simulink library "Tire_MFSwift"  (R2019a)
settings: Solver=VariableStepAuto  StartTime=0.0  StopTime=10.0  RelTol=1e-3
undefined symbols (not defined in the file): Left, UNLOADED_RADIUS, Vehicle, VERTICAL_DAMPING, VERTICAL_STIFFNESS, Visual, X, Y, Z
libraries: nesl_utility x24, sm_lib x15, mfswift_simscape_library x2, Delft_Tyre_dtlib x1, TireBody_Models x1, sm_car_lib x1, $bdroot x1
(part 2 of 2)

== system Tire_MFSwift/CPI Tire/Tire and Force ==
  Inertia : sm_lib/Body Elements/Solid  InertiaType=Custom  Mass=mass  MassUnits=kg  CenterOfMass=[0 0 0]  CenterOfMassUnits=m  MomentsOfInertia=[Imat(1,1) Imat(2,2) Imat(3,3)]  MomentsOfInertiaUnits=kg*m^2  ProductsOfInertia=[0 0 0]  ProductsOfInertiaUnits=kg*m^2  BasedOnType=Density  Density=1000  DensityUnits=kg/(m^3)  DoExposeReferenceFrame=on  SerializedFrames=<Frames/>  GraphicType=FromGeometry  MarkerShape=Sphere  MarkerSize=10  MarkerSizeUnits=m  GraphicVisPropType=SimpleVisualProperties  GraphicDiffuseColor=[0.2 0.8 1.0]  GraphicSpecularColor=[0.5 0.5 0.5 1.0]  GraphicAmbientColor=[0.15 0.15 0.15 1.0]  GraphicEmissiveColor=[0.0 0.0 0.0 1.0]  GraphicShininess=75  GraphicOpacity=1.0  GeometryShape=Cylinder  RectangleSize=[1 1]  RectangleSizeUnits=m  BrickDimensions=[3 1 0.5]  BrickDimensionUnits=m  CylinderRadius=0.001  CylinderRadiusUnits=m  CylinderLength=0.001  CylinderLengthUnits=m  SphereRadius=0.001  SphereRadiusUnits=m  EllipsoidRadii=[1 1 1]  EllipsoidRadiiUnits=m  ExtrusionCrossSection=[1 1; -1 1; -1 -1; 1 -1]  ExtrusionCrossSectionUnits=m  ExtrusionLength=1  ExtrusionLengthUnits=m  PolygonNumSides=3  PolygonOuterRadius=1  PolygonOuterRadiusUnits=m  ExtGeomFileType=STEP  ExtGeomFileName=.\CadImportFiles\Tire.STL  ExtGeomFileUnits=mm  RevolutionCrossSection=[1 1; 1 -1; 2 -1; 2 1]  RevolutionCrossSectionUnits=m  RevolutionExtent=Full  RevolutionAngle=180  RevolutionAngleUnits=deg
  Rim : sm_lib/Body Elements/Solid  InertiaType=Custom  Mass=0  MassUnits=kg  CenterOfMass=[0 0 0]  CenterOfMassUnits=m  MomentsOfInertia=[0 0 0]  MomentsOfInertiaUnits=kg*m^2  ProductsOfInertia=[0 0 0]  ProductsOfInertiaUnits=kg*m^2  BasedOnType=Density  Density=1000  DensityUnits=kg/(m^3)  DoExposeReferenceFrame=on  SerializedFrames=<Frames/>  GraphicType=FromGeometry  MarkerShape=Sphere  MarkerSize=10  MarkerSizeUnits=m  GraphicVisPropType=SimpleVisualProperties  GraphicDiffuseColor=clr_rim_cfl  GraphicSpecularColor=[0.5 0.5 0.5 1.0]  GraphicAmbientColor=[0.15 0.15 0.15 1.0]  GraphicEmissiveColor=[0.0 0.0 0.0 1.0]  GraphicShininess=75  GraphicOpacity=opc_rim_cfl  GeometryShape=RegularExtrusion  RectangleSize=[1 1]  RectangleSizeUnits=m  BrickDimensions=[1 1 1]  BrickDimensionUnits=m  CylinderRadius=1  CylinderRadiusUnits=m  CylinderLength=1  CylinderLengthUnits=m  SphereRadius=1  SphereRadiusUnits=m  EllipsoidRadii=[1 1 1]  EllipsoidRadiiUnits=m  ExtrusionCrossSection=[1 1; -1 1; -1 -1; 1 -1]  ExtrusionCrossSectionUnits=m  ExtrusionLength=width*0.1  ExtrusionLengthUnits=m  PolygonNumSides=5  PolygonOuterRadius=rim_radius  PolygonOuterRadiusUnits=m  ExtGeomFileType=STL  ExtGeomFileName=Rim.STL  ExtGeomFileUnits=mm  RevolutionCrossSection=[1 1; 1 -1; 2 -1; 2 1]  RevolutionCrossSectionUnits=m  RevolutionExtent=Full  RevolutionAngle=180  RevolutionAngleUnits=deg
  Tire : sm_lib/Body Elements/Solid  InertiaType=Custom  Mass=0  MassUnits=kg  CenterOfMass=[0 0 0]  CenterOfMassUnits=m  MomentsOfInertia=[0 0 0]  MomentsOfInertiaUnits=kg*m^2  ProductsOfInertia=[0 0 0]  ProductsOfInertiaUnits=kg*m^2  BasedOnType=Density  Density=1000  DensityUnits=kg/(m^3)  DoExposeReferenceFrame=on  SerializedFrames=<Frames/>  GraphicType=FromGeometry  MarkerShape=Sphere  MarkerSize=10  MarkerSizeUnits=m  GraphicVisPropType=SimpleVisualProperties  GraphicDiffuseColor=clr_tyre_cfl  GraphicSpecularColor=[0.5 0.5 0.5 1.0]  GraphicAmbientColor=[0.15 0.15 0.15 1.0]  GraphicEmissiveColor=[0.0 0.0 0.0 1.0]  GraphicShininess=75  GraphicOpacity=opc_tyre_cfl  GeometryShape=GeneralSolidOfRevolution  RectangleSize=[1 1]  RectangleSizeUnits=m  BrickDimensions=[1 1 1]  BrickDimensionUnits=m  CylinderRadius=1  CylinderRadiusUnits=m  CylinderLength=1  CylinderLengthUnits=m  SphereRadius=1  SphereRadiusUnits=m  EllipsoidRadii=[1 1 1]  EllipsoidRadiiUnits=m  ExtrusionCrossSection=[1 1; -1 1; -1 -1; 1 -1]  ExtrusionCrossSectionUnits=m  ExtrusionLength=1  ExtrusionLengthUnits=m  PolygonNumSides=3  PolygonOuterRadius=1  PolygonOuterRadiusUnits=m  ExtGeomFileType=STL  ExtGeomFileName=Tire.STL  ExtGeomFileUnits=mm  RevolutionCrossSection="[1  0.5; rim_radius/radius 0.5; rim_radius/radius -0.5; 1 -0.5].*[radius  width]"  RevolutionCrossSectionUnits=m  RevolutionExtent=Full  RevolutionAngle=180  RevolutionAngleUnits=deg
  Transform Geometry : sm_lib/Frames and Transforms/Rigid Transform  TranslationMethod=StandardAxis  TranslationStandardOffset=0  TranslationLengthUnit=m  TranslationStandardAxis=+Y  TranslationCartesianOffset=[0 0 0]  TranslationROffset=0  TranslationROffsetUnits=m  TranslationZOffset=0  TranslationZOffsetUnits=m  TranslationThetaOffset=0  TranslationThetaOffsetUnits=deg  RotationMethod=StandardAxis  RotationAngleUnits=deg  RotationStandardAxis=+X  RotationAngle=-90  RotationArbitraryAxis=[0 0 1]  FollAlignAxisA=+X  BaseAlignAxisA=+Y  FollAlignAxisB=+Y  BaseAlignAxisB=+Z  RotationSequenceAxes=FollowerAxes  RotationSequence=XYX  RotationSequenceAngles=[0 0 0]  RotationSequenceAnglesUnits=deg  RotationMatrix=[1 0 0; 0 1 0; 0 0 1]
  Transform Spin Axis : sm_lib/Frames and Transforms/Rigid Transform  TranslationMethod=None  TranslationStandardOffset=0  TranslationLengthUnit=m  TranslationStandardAxis=+Z  TranslationCartesianOffset=[0 0 0]  TranslationROffset=0  TranslationROffsetUnits=m  TranslationZOffset=0  TranslationZOffsetUnits=m  TranslationThetaOffset=0  TranslationThetaOffsetUnits=deg  RotationMethod=StandardAxis  RotationAngleUnits=deg  RotationStandardAxis=-X  RotationAngle=90  RotationArbitraryAxis=[0 0 1]  FollAlignAxisA=+X  BaseAlignAxisA=+Y  FollAlignAxisB=+Y  BaseAlignAxisB=+Z  RotationSequenceAxes=FollowerAxes  RotationSequence=XYX  RotationSequenceAngles=[0 0 0]  RotationSequenceAnglesUnits=deg  RotationMatrix=[1 0 0; 0 1 0; 0 0 1]
  B : PMIOPort  Side=Left
  connections:
  Transform Spin Axis/RConn1 -- B/RConn1
  Tire/RConn1 -- Transform Geometry/RConn1 -- Inertia/RConn1 -- Rim/RConn1
  Transform Spin Axis/LConn1 -- Transform Geometry/LConn1

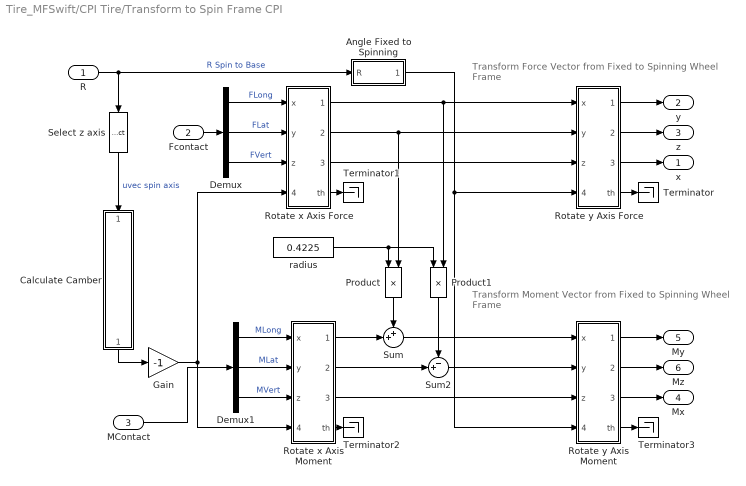
== system Tire_MFSwift/CPI Tire/Transform to Spin Frame CPI ==
  note: Transform Moment Vector from Fixed
      | to Spinning Wheel Frame
  note: Transform Force Vector from Fixed
      | to Spinning Wheel Frame
  R : Inport
  Fcontact : Inport  Port=2
  MContact : Inport  Port=3
  Angle Fixed to Spinning : Subsystem
  Calculate Camber : Subsystem
  Demux : Demux  Outputs=3
  Demux1 : Demux  Outputs=3
  Gain : Gain  Gain=-1
  Product : Product
  Product1 : Product
  Rotate x Axis Force : Subsystem
  Rotate x Axis Moment : Subsystem
  Rotate y Axis Force : Subsystem
  Rotate y Axis Moment : Subsystem
  Select z axis : Selector  NumberOfDimensions=2  InputPortWidth=2  IndexOptions=Index vector (dialog),Index vector (dialog)  Indices=[1 2 3],3  OutputSizes=1,1
  Sum : Sum  Inputs=++|
  Sum2 : Sum  Inputs=-+|
  Terminator{,1..3} (4 alike) : Terminator
  radius : Constant  Value=0.4225
  x : Outport
  y : Outport  Port=2
  z : Outport  Port=3
  Mx : Outport  Port=4
  My : Outport  Port=5
  Mz : Outport  Port=6
  wires:
  R/1 -> Select z axis/1, Angle Fixed to Spinning/1(R)  "R Spin to Base"
  Angle Fixed to Spinning/1(rotang) -> Rotate y Axis Moment/4(theta), Rotate y Axis Force/4(theta)
  Rotate y Axis Moment/1(x rot) -> My/1
  Rotate y Axis Moment/2(y rot) -> Mz/1
  Rotate x Axis Moment/1(x rot) -> Sum/2
  Rotate x Axis Force/1(x rot) -> Product1/2, Rotate y Axis Force/1(x)
  Rotate y Axis Force/1(x rot) -> y/1
  Rotate y Axis Force/2(y rot) -> z/1
  Select z axis/1 -> Calculate Camber/1(uvec spin axis)  "uvec spin axis"
  Demux/1 -> Rotate x Axis Force/1(x)  "FLong"
  Demux/3 -> Rotate x Axis Force/3(z)  "FVert"
  Calculate Camber/1(Camber) -> Gain/1
  Demux1/3 -> Rotate x Axis Moment/3(z)  "MVert"
  Demux1/1 -> Rotate x Axis Moment/1(x)  "MLong"
  Demux1/2 -> Rotate x Axis Moment/2(y)  "MLat"
  Product/1 -> Sum/1
  radius/1 -> Product1/1, Product/1
  Rotate x Axis Force/3(z rot) -> Rotate y Axis Force/3(z)
  Product1/1 -> Sum2/1
  Demux/2 -> Rotate x Axis Force/2(y)  "FLat"
  Rotate x Axis Force/2(y rot) -> Rotate y Axis Force/2(y), Product/2
  Rotate y Axis Force/3(z rot) -> x/1
  Rotate y Axis Force/4(th) -> Terminator/1
  Rotate x Axis Force/4(th) -> Terminator1/1
  Rotate x Axis Moment/2(y rot) -> Sum2/2
  Rotate x Axis Moment/4(th) -> Terminator2/1
  Rotate y Axis Moment/3(z rot) -> Mx/1
  Rotate y Axis Moment/4(th) -> Terminator3/1
  Sum2/1 -> Rotate y Axis Moment/2(y)
  Sum/1 -> Rotate y Axis Moment/1(x)
  Rotate x Axis Moment/3(z rot) -> Rotate y Axis Moment/3(z)
  Gain/1 -> Rotate x Axis Force/4(theta), Rotate x Axis Moment/4(theta)
  Fcontact/1 -> Demux/1
  MContact/1 -> Demux1/1

== system Tire_MFSwift/CPI Tire/Vertical Force ==
  camber : Inport
  h : Inport  Port=2
  vz : Inport  Port=3
  gz : Inport  Port=4
  Constant1 : Constant  Value=UNLOADED_RADIUS
  Cos : Trigonometry  Operator=cos
  Damping Force : Subsystem
  Product : Product
  Subtract : Sum  Inputs=+-
  Sum : Sum  Inputs=|+-
  Sum1 : Sum  Inputs=|+-
  Tire Vertical Stiffness : Lookup_n-D  NumberOfTableDimensions=1  BreakpointsForDimension1=[-1 0 0.1]  Table=[VERTICAL_STIFFNESS 0 0]  InternalRulePriority=Speed  RndMeth=Simplest  InputSameDT=on
  Fvert : Outport
  wires:
  h/1 -> Subtract/1
  Sum1/1 -> Fvert/1
  camber/1 -> Cos/1
  gz/1 -> Sum/2
  Cos/1 -> Product/2
  vz/1 -> Damping Force/2(vz)
  Subtract/1 -> Sum/1
  Damping Force/1(Fz d) -> Sum1/2
  Product/1 -> Subtract/2
  Sum/1 -> Tire Vertical Stiffness/1
  Constant1/1 -> Product/1
  Tire Vertical Stiffness/1 -> Damping Force/1(Fz k), Sum1/1

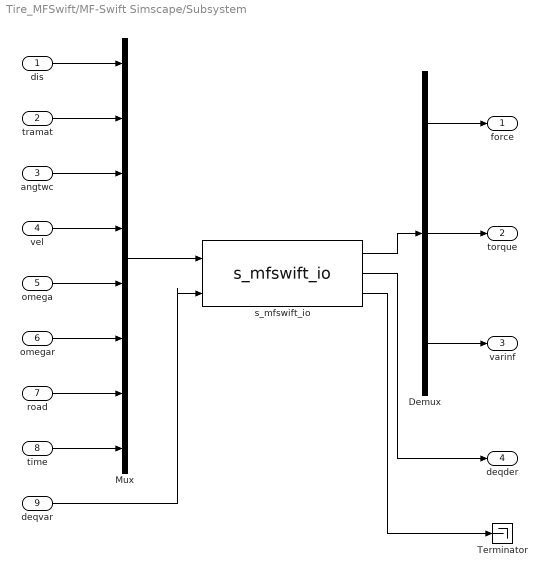
== system Tire_MFSwift/MF-Swift Simscape/Subsystem ==
  dis : Inport
  tramat : Inport  Port=2
  angtwc : Inport  Port=3
  vel : Inport  Port=4
  omega : Inport  Port=5
  omegar : Inport  Port=6
  road : Inport  Port=7
  time : Inport  Port=8
  deqvar : Inport  Port=9
  Demux : Demux  Outputs=[3 3 60]
  Mux : Mux  Inputs=[3 9 1 3 3 1 20 1]
  Terminator : Terminator
  s_mfswift_io : S-Function  FunctionName=s_mfswift_io  Parameters=SParameter1, SParameter2, SParameter3, SParameter4, SParameter5,SParameter6,SParameter7  SFunctionDeploymentMode=off  EnableBusSupport=off  mask(Legacy Function){SFunctionSpec=tyre_outputs(void **work1, int32 p2, int16 p4[8], double u1[41], double u2[40], int16 work2[1], double work3[1], double y1[66], double y2[40], int16 y3[1]), SParameter1=iswtch, SParameter2=idtyre, SParameter3=typarr, SParameter4=uint8([tyreSimulationMode 0]), SParameter5=uint8([tyreTargetFile 0]), SParameter6=uint8([tyreTemplateMakefile 0]), SParameter7=roadfile, ShowSpec=off}
      mask prompts: SParameter1 "P1: iswtch"; SParameter2 "P2: idtyre"; SParameter3 "P3: typarr"; SParameter4 "P4: simulation mode"; SParameter5 "P5: target file"; SParameter6 "P6: template makefile"; SParameter7 "P7: road file name"; ShowSpec "Display function specification"
      mask help:
      | This block allows you to call the legacy functions specified by the following Legacy Code Tool definition:
      | def.SFunctionName = 's_mfswift_io';
      | def.OutputFcnSpec = 'tyre_outputs(void **work1, int32 p2, int16 p4[8], double u1[41], double u2[40], int16 work2[1], double work3[1], double y1[66], double y2[40], int16 y3[1])';
      | def.StartFcnSpec = 'tyre_start(void **work1, int32 p1, int32 p2, double p3[300], int16 p4[8], uint8 p5[], int16 work2[1], double work3[1])';
      | def.TerminateFcnSpec = 'tyre_terminate(void **work1, int32 p2, int16 p4[8], int16 work2[1])';
      | def.HeaderFiles = {'tyremain.h', 'mfs_dtemsg.h'};
      | def.SourceFiles = {'dtemsg.c', 'console_writer.c'};
      | def.HostLibFiles = {'s_mfswift_io_impld.lib'};
      | def.TargetLibFiles = {'mfs_platform_generic_r2009a_ds1006.lib', 'mfs_kernel_r2009a_ds1006.lib', 'mfs_callback_r2009a_ds1006.lib', 'mfs_generic_r2009a_ds1006.lib', 'mfs_utilities_system_r2009a_ds1006.lib', 'mfs_platform_license_flexlm_r2009a_ds1006.lib', 'mfs_platform_license_stub_r2009a_ds1006.lib', 'mfs_log_r2009a_ds1006.lib'};
      | def.IncPaths = {'../headers'};
      | def.SrcPaths = {'../sources'};
      | def.LibPaths = {'../libraries/windows_win64', '../libraries/dSPACE_ds1006'};
      mask Help: <p>This block was generated automatically by the Legacy Code Tool. For detailed help on this tool, call<a href="matlab:legacy_code('help')"> legacy_code('help')</a>.</p>
      mask Callback ShowSpec:
      | if strcmp(get_param(gcbh, 'ShowSpec'), 'on')
      |   set_param(gcbh, 'MaskDisplay', sprintf('fprintf(''%s'');', get_param(gcbh, 'SFunctionSpec')));
      | else
      |   set_param(gcbh, 'MaskDisplay', sprintf('fprintf(''%s'');', get_param(gcbh, 'FunctionName')));
      | end
      mask Display: fprintf('s_mfswift_io');
  force : Outport  VectorParamsAs1DForOutWhenUnconnected=on
  torque : Outport  Port=2  VectorParamsAs1DForOutWhenUnconnected=on
  varinf : Outport  Port=3  VectorParamsAs1DForOutWhenUnconnected=on
  deqder : Outport  Port=4  VectorParamsAs1DForOutWhenUnconnected=on
  wires:
  tramat/1 -> Mux/2
  angtwc/1 -> Mux/3
  vel/1 -> Mux/4
  omega/1 -> Mux/5
  omegar/1 -> Mux/6
  road/1 -> Mux/7
  dis/1 -> Mux/1
  Demux/2 -> torque/1
  Demux/1 -> force/1
  Demux/3 -> varinf/1
  Mux/1 -> s_mfswift_io/1
  s_mfswift_io/1 -> Demux/1
  s_mfswift_io/2 -> deqder/1
  deqvar/1 -> s_mfswift_io/2
  time/1 -> Mux/8
  s_mfswift_io/3 -> Terminator/1

== system Tire_MFSwift/MF-Swift Simscape/add signal names ==
  In1 : Inport
  Added for future extension : Terminator
  Bus Creator : BusCreator  Inputs=40
  Demux1 : Demux  Outputs=[ones(1,40) -1]
  Out1 : Outport  VectorParamsAs1DForOutWhenUnconnected=on
  wires:
  Demux1/41 -> Added for future extension/1
  Demux1/40 -> Bus Creator/40  "eff_plane_banking"
  Demux1/39 -> Bus Creator/39  "eff_plane_curvature"
  Demux1/38 -> Bus Creator/38  "eff_plane_angle"
  Demux1/37 -> Bus Creator/37  "eff_plane_height"
  Demux1/36 -> Bus Creator/36  "nz"
  Demux1/35 -> Bus Creator/35  "ny"
  Demux1/34 -> Bus Creator/34  "nx"
  Demux1/33 -> Bus Creator/33  "zcp"
  Demux1/32 -> Bus Creator/32  "ycp"
  Demux1/31 -> Bus Creator/31  "xcp"
  Demux1/30 -> Bus Creator/30  "_e30"
  Demux1/29 -> Bus Creator/29  "_e29"
  Demux1/28 -> Bus Creator/28  "travelled_distance"
  Demux1/27 -> Bus Creator/27  "_e27"
  Demux1/26 -> Bus Creator/26  "_e26"
  Demux1/25 -> Bus Creator/25  "_e25"
  Demux1/24 -> Bus Creator/24  "psidot"
  Demux1/23 -> Bus Creator/23  "Vz"
  Demux1/22 -> Bus Creator/22  "Vsy"
  Demux1/21 -> Bus Creator/21  "Vsx"
  Demux1/20 -> Bus Creator/20  "relaxation_length_y"
  Demux1/19 -> Bus Creator/19  "relaxation_length_x"
  Demux1/18 -> Bus Creator/18  "mu_y"
  Demux1/17 -> Bus Creator/17  "mu_x"
  Demux1/16 -> Bus Creator/16  "pneumatic_trail"
  Demux1/15 -> Bus Creator/15  "contact_length"
  Demux1/14 -> Bus Creator/14  "vertical_deflection"
  Demux1/13 -> Bus Creator/13  "effective_rolling_radius"
  Demux1/12 -> Bus Creator/12  "_e12"
  Demux1/11 -> Bus Creator/11  "Vx"
  Demux1/10 -> Bus Creator/10  "turn_slip"
  Demux1/9 -> Bus Creator/9  "inclination_angle"
  Demux1/8 -> Bus Creator/8  "side_slip_angle"
  Demux1/7 -> Bus Creator/7  "longitudinal_slip"
  Demux1/6 -> Bus Creator/6  "Mz"
  Demux1/5 -> Bus Creator/5  "My"
  Demux1/4 -> Bus Creator/4  "Mx"
  Demux1/3 -> Bus Creator/3  "Fz"
  Demux1/2 -> Bus Creator/2  "Fy"
  Demux1/1 -> Bus Creator/1  "Fx"
  Bus Creator/1 -> Out1/1  "varinf"
  In1/1 -> Demux1/1

== system Tire_MFSwift/MFSwift/Road Inputs ==
  note: 1) Only subsystems can be added as variant choices at this level
      | 2) Blocks cannot be connected at this level as connectivity is
      | automatically determined at simulation, based on the active variant
  RdBus : Inport
  External Road : Subsystem  VariantControl=ExternalRoad
  Non-moving road : mfswift_simscape_library/Non-moving road  VariantControl=NonMoving  dummy=off
  Test Rig Post : Subsystem  VariantControl=TestRigPost
  road : Outport

== system Tire_MFSwift/CPI Tire/Sensing Wheel Fixed Frame/Ang Velocity Vector ==
  Mux : Mux  Inputs=3
  PS-Simulink Converter1 : nesl_utility/PS-Simulink Converter  PhysicalDomain=network_engine_domain  SubClassName=ps_output  LeftPortType=input  RightPortType=output  PseudoPeriodic=off  Frequencies=[]  Unit=1  AffineConversion=off
  PS-Simulink Converter2 : nesl_utility/PS-Simulink Converter  PhysicalDomain=network_engine_domain  SubClassName=ps_output  LeftPortType=input  RightPortType=output  PseudoPeriodic=off  Frequencies=[]  Unit=1  AffineConversion=off
  PS-Simulink Converter3 : nesl_utility/PS-Simulink Converter  PhysicalDomain=network_engine_domain  SubClassName=ps_output  LeftPortType=input  RightPortType=output  PseudoPeriodic=off  Frequencies=[]  Unit=rad/s  AffineConversion=off
  Scope : Scope
  wx : PMIOPort  Side=Left
  wy : PMIOPort  Port=2  Side=Left
  wz : PMIOPort  Port=3  Side=Left
  wxyz : Outport
  wires:
  PS-Simulink Converter1/1 -> Mux/1
  PS-Simulink Converter3/1 -> Mux/3
  PS-Simulink Converter2/1 -> Mux/2
  Mux/1 -> wxyz/1, Scope/1
  connections:
  PS-Simulink Converter2/LConn1 -- wy/RConn1
  wx/RConn1 -- PS-Simulink Converter1/LConn1
  wz/RConn1 -- PS-Simulink Converter3/LConn1

== system Tire_MFSwift/CPI Tire/Sensing Wheel Fixed Frame/Calculate Camber ==
  uvec spin axis : Inport
  Demux : Demux  Outputs=3
  Mux : Mux  Inputs=2
  Trigonometric Function1 : Trigonometry  Operator=atan2
  magnitude : Fcn  Expr=sqrt(u(1)*u(1)+u(2)*u(2))
  Camber : Outport
  wires:
  Demux/1 -> Mux/1
  uvec spin axis/1 -> Demux/1
  Trigonometric Function1/1 -> Camber/1
  Demux/3 -> Trigonometric Function1/1
  Mux/1 -> magnitude/1
  magnitude/1 -> Trigonometric Function1/2
  Demux/2 -> Mux/2

== system Tire_MFSwift/CPI Tire/Sensing Wheel Fixed Frame/Get uvec Yaw axis ==
  note: Make Unit Vector
  note: Obtain unit vector along vertical axis within tire plane (wheel yaw axis)
      | (World Z vector [0 0 1])  -  (z-component of unit vector along wheel spin axis)
      | normalize ([0 0 1] - ([0 0 1].*uvec spin axis)*uvec spin axis)
  zf : Inport
  Add : Sum
  Constant : Constant
  Demux : Demux  Outputs=3
  Divide : Product  Inputs=*/
  Gain2 : Gain  Gain=-1
  Mult : Product  Inputs=**
  Mult1 : Product  Inputs=**
  Mult2 : Product  Inputs=**
  Mux1 : Mux  Inputs=3
  magnitude : Fcn  Expr=sqrt(u(1)*u(1)+u(2)*u(2)+u(3)*u(3))
  u : Outport
  wires:
  Add/1 -> Mux1/3
  Demux/2 -> Mult1/1
  Mux1/1 -> magnitude/1, Divide/1  "u0"
  Mult2/1 -> Add/1
  Demux/1 -> Mult/1
  zf/1 -> Demux/1
  Demux/3 -> Gain2/1, Mult2/1
  Gain2/1 -> Mult2/2, Mult1/2, Mult/2
  Mult1/1 -> Mux1/2
  Mult/1 -> Mux1/1
  Constant/1 -> Add/2
  Divide/1 -> u/1
  magnitude/1 -> Divide/2

== system Tire_MFSwift/CPI Tire/Sensing Wheel Fixed Frame/Project onto Road Plane ==
  note: Normalize to create a unit vector
  note: Create unit vector in lateral direction from wheel on ground plane.
      |
      | This computation projects input vector v (along the wheel spin axis) onto the plane normal to the z axis.
  v : Inport
  Constant : Constant  Value=0
  Demux : Demux  Outputs=3
  Divide : Product  Inputs=*/
  Mux1 : Mux  Inputs=3
  Terminator : Terminator
  magnitude : Fcn  Expr=sqrt(u(1)*u(1)+u(2)*u(2))
  v proj : Outport
  wires:
  Mux1/1 -> Divide/1, magnitude/1
  Demux/2 -> Mux1/2
  Demux/1 -> Mux1/1
  Constant/1 -> Mux1/3
  Demux/3 -> Terminator/1
  v/1 -> Demux/1
  Divide/1 -> v proj/1
  magnitude/1 -> Divide/2

== system Tire_MFSwift/CPI Tire/Sensing Wheel Fixed Frame/Rot -90 deg about Z ==
  v : Inport
  Demux : Demux  Outputs=3
  Gain : Gain  Gain=-1
  Mux1 : Mux  Inputs=3
  v rot -z : Outport
  wires:
  Demux/1 -> Gain/1
  Mux1/1 -> v rot -z/1
  Demux/3 -> Mux1/3
  Gain/1 -> Mux1/2
  Demux/2 -> Mux1/1
  v/1 -> Demux/1

== system Tire_MFSwift/CPI Tire/Sensing Wheel Fixed Frame/Velocity Vector ==
  Mux : Mux  Inputs=3
  PS-Simulink Converter1 : nesl_utility/PS-Simulink Converter  PhysicalDomain=network_engine_domain  SubClassName=ps_output  LeftPortType=input  RightPortType=output  PseudoPeriodic=off  Frequencies=[]  Unit=1  AffineConversion=off
  PS-Simulink Converter2 : nesl_utility/PS-Simulink Converter  PhysicalDomain=network_engine_domain  SubClassName=ps_output  LeftPortType=input  RightPortType=output  PseudoPeriodic=off  Frequencies=[]  Unit=1  AffineConversion=off
  PS-Simulink Converter3 : nesl_utility/PS-Simulink Converter  PhysicalDomain=network_engine_domain  SubClassName=ps_output  LeftPortType=input  RightPortType=output  PseudoPeriodic=off  Frequencies=[]  Unit=1  AffineConversion=off
  vx : PMIOPort  Side=Left
  vy : PMIOPort  Port=2  Side=Left
  vz : PMIOPort  Port=3  Side=Left
  vxyz : Outport
  wires:
  PS-Simulink Converter1/1 -> Mux/1
  PS-Simulink Converter3/1 -> Mux/3
  PS-Simulink Converter2/1 -> Mux/2
  Mux/1 -> vxyz/1
  connections:
  PS-Simulink Converter2/LConn1 -- vy/RConn1
  vx/RConn1 -- PS-Simulink Converter1/LConn1
  vz/RConn1 -- PS-Simulink Converter3/LConn1

== system Tire_MFSwift/CPI Tire/Transform to Spin Frame CPI/Angle Fixed to Spinning ==
  R : Inport
  Atan2 : Trigonometry  Operator=atan2
  Demux1 : Demux  Outputs=3
  Get uvec Yaw axis : Subsystem
  Multiply : Product  Inputs=**  Multiplication=Matrix(*)
  Select z axis : Selector  NumberOfDimensions=2  InputPortWidth=2  IndexOptions=Index vector (dialog),Index vector (dialog)  Indices=[1 2 3],3  OutputSizes=1,1
  Terminator : Terminator
  Transpose : Math  Operator=transpose  SaturateOnIntegerOverflow=on
  rotang : Outport
  wires:
  Demux1/2 -> Atan2/1
  Get uvec Yaw axis/1(u) -> Multiply/2  "Yaw vec Base"
  Demux1/1 -> Atan2/2
  Demux1/3 -> Terminator/1
  Select z axis/1 -> Get uvec Yaw axis/1(zf)  "uvec spin axis"
  R/1 -> Select z axis/1, Transpose/1
  Atan2/1 -> rotang/1
  Multiply/1 -> Demux1/1  "yaw vec spin frame"
  Transpose/1 -> Multiply/1  "R Base 2 Spin Frame"

== system Tire_MFSwift/CPI Tire/Transform to Spin Frame CPI/Calculate Camber ==
  uvec spin axis : Inport
  Demux : Demux  Outputs=3
  Mux : Mux  Inputs=2
  Trigonometric Function1 : Trigonometry  Operator=atan2
  magnitude : Fcn  Expr=sqrt(u(1)*u(1)+u(2)*u(2))
  Camber : Outport
  wires:
  Demux/2 -> Mux/2
  magnitude/1 -> Trigonometric Function1/2
  Mux/1 -> magnitude/1
  Demux/3 -> Trigonometric Function1/1
  Trigonometric Function1/1 -> Camber/1
  uvec spin axis/1 -> Demux/1
  Demux/1 -> Mux/1

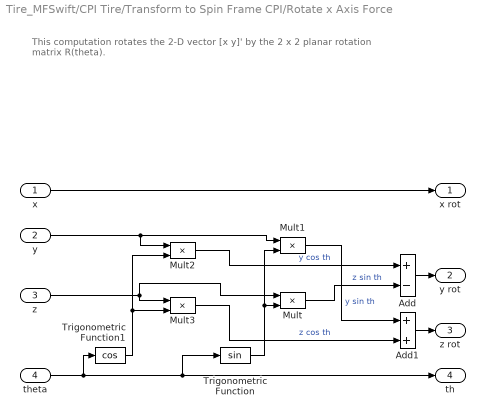
== system Tire_MFSwift/CPI Tire/Transform to Spin Frame CPI/Rotate x Axis Force ==
  note: This computation rotates the 2-D vector [x y]' by the 2 x 2
      | planar rotation matrix R(theta).
  x : Inport
  y : Inport  Port=2
  z : Inport  Port=3
  theta : Inport  Port=4
  Add : Sum  Inputs=+-
  Add1 : Sum
  Mult{,1..3} (4 alike) : Product  Inputs=**
  Trigonometric Function : Trigonometry
  Trigonometric Function1 : Trigonometry  Operator=cos
  x rot : Outport
  y rot : Outport  Port=2
  z rot : Outport  Port=3
  th : Outport  Port=4
  wires:
  theta/1 -> th/1, Trigonometric Function/1, Trigonometric Function1/1
  y/1 -> Mult1/1, Mult2/1
  z/1 -> Mult3/1, Mult/1
  Trigonometric Function1/1 -> Mult2/2, Mult3/2
  Trigonometric Function/1 -> Mult1/2, Mult/2
  Mult2/1 -> Add/1  "y cos th"
  Add/1 -> y rot/1
  Mult3/1 -> Add1/2  "z cos th"
  Add1/1 -> z rot/1
  Mult/1 -> Add/2  "z sin th"
  Mult1/1 -> Add1/1  "y sin th"
  x/1 -> x rot/1

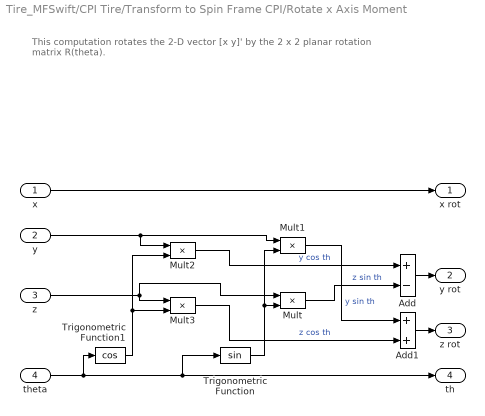
== system Tire_MFSwift/CPI Tire/Transform to Spin Frame CPI/Rotate x Axis Moment ==
  note: This computation rotates the 2-D vector [x y]' by the 2 x 2
      | planar rotation matrix R(theta).
  x : Inport
  y : Inport  Port=2
  z : Inport  Port=3
  theta : Inport  Port=4
  Add : Sum  Inputs=+-
  Add1 : Sum
  Mult{,1..3} (4 alike) : Product  Inputs=**
  Trigonometric Function : Trigonometry
  Trigonometric Function1 : Trigonometry  Operator=cos
  x rot : Outport
  y rot : Outport  Port=2
  z rot : Outport  Port=3
  th : Outport  Port=4
  wires:
  x/1 -> x rot/1
  Mult1/1 -> Add1/1  "y sin th"
  Mult/1 -> Add/2  "z sin th"
  Add1/1 -> z rot/1
  Mult3/1 -> Add1/2  "z cos th"
  Add/1 -> y rot/1
  Mult2/1 -> Add/1  "y cos th"
  Trigonometric Function/1 -> Mult/2, Mult1/2
  Trigonometric Function1/1 -> Mult3/2, Mult2/2
  z/1 -> Mult/1, Mult3/1
  y/1 -> Mult2/1, Mult1/1
  theta/1 -> Trigonometric Function1/1, Trigonometric Function/1, th/1

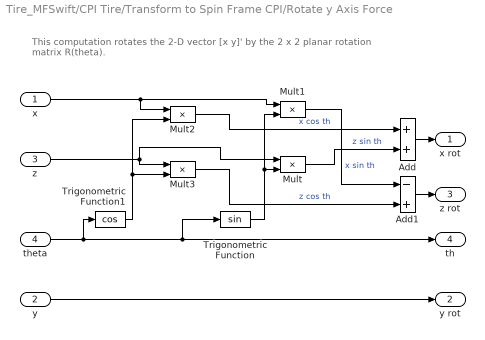
== system Tire_MFSwift/CPI Tire/Transform to Spin Frame CPI/Rotate y Axis Force ==
  note: This computation rotates the 2-D vector [x y]' by the 2 x 2
      | planar rotation matrix R(theta).
  x : Inport
  y : Inport  Port=2
  z : Inport  Port=3
  theta : Inport  Port=4
  Add : Sum
  Add1 : Sum  Inputs=-+
  Mult{,1..3} (4 alike) : Product  Inputs=**
  Trigonometric Function : Trigonometry
  Trigonometric Function1 : Trigonometry  Operator=cos
  x rot : Outport
  y rot : Outport  Port=2
  z rot : Outport  Port=3
  th : Outport  Port=4
  wires:
  Mult1/1 -> Add1/1  "x sin th"
  Mult/1 -> Add/2  "z sin th"
  Add1/1 -> z rot/1
  Mult3/1 -> Add1/2  "z cos th"
  Add/1 -> x rot/1
  Mult2/1 -> Add/1  "x cos th"
  Trigonometric Function/1 -> Mult/2, Mult1/2
  Trigonometric Function1/1 -> Mult3/2, Mult2/2
  z/1 -> Mult/1, Mult3/1
  x/1 -> Mult2/1, Mult1/1
  theta/1 -> Trigonometric Function1/1, th/1, Trigonometric Function/1
  y/1 -> y rot/1

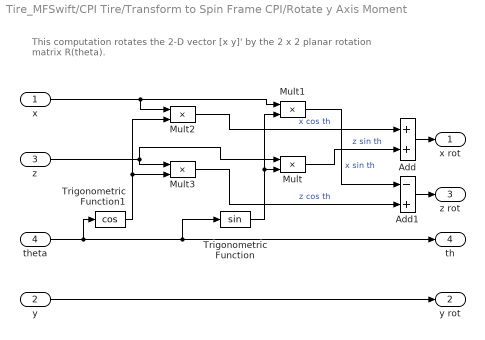
== system Tire_MFSwift/CPI Tire/Transform to Spin Frame CPI/Rotate y Axis Moment ==
  note: This computation rotates the 2-D vector [x y]' by the 2 x 2
      | planar rotation matrix R(theta).
  x : Inport
  y : Inport  Port=2
  z : Inport  Port=3
  theta : Inport  Port=4
  Add : Sum
  Add1 : Sum  Inputs=-+
  Mult{,1..3} (4 alike) : Product  Inputs=**
  Trigonometric Function : Trigonometry
  Trigonometric Function1 : Trigonometry  Operator=cos
  x rot : Outport
  y rot : Outport  Port=2
  z rot : Outport  Port=3
  th : Outport  Port=4
  wires:
  y/1 -> y rot/1
  theta/1 -> Trigonometric Function/1, th/1, Trigonometric Function1/1
  x/1 -> Mult1/1, Mult2/1
  z/1 -> Mult3/1, Mult/1
  Trigonometric Function1/1 -> Mult2/2, Mult3/2
  Trigonometric Function/1 -> Mult1/2, Mult/2
  Mult2/1 -> Add/1  "x cos th"
  Add/1 -> x rot/1
  Mult3/1 -> Add1/2  "z cos th"
  Add1/1 -> z rot/1
  Mult/1 -> Add/2  "z sin th"
  Mult1/1 -> Add1/1  "x sin th"

== system Tire_MFSwift/CPI Tire/Vertical Force/Damping Force ==
  note: Apply damping only when stiffness force >0
  Fz k : Inport
  vz : Inport  Port=2
  Constant : Constant  Value=0
  Constant1 : Constant  Value=VERTICAL_DAMPING
  Product : Product
  Switch : Switch  Criteria=u2 > Threshold  ZeroCross=off
  Fz d : Outport
  wires:
  Constant1/1 -> Product/2
  Constant/1 -> Switch/3
  Switch/1 -> Fz d/1
  Fz k/1 -> Switch/2
  Product/1 -> Switch/1
  vz/1 -> Product/1

== system Tire_MFSwift/MFSwift/Road Inputs/External Road ==
  RdBus : Inport
  Bus Creator : BusCreator  Commented=on  Inputs=3
  Bus Selector : BusSelector  OutputSignals=gz,uvec,TyreScaling
  Constant1 : Constant  Commented=on  Value=[0 0 0]
  Constant2 : Constant  Commented=on  Value=0
  Constant3 : Constant  Value=[0 0]
  Constant4 : Constant  Value=[0 0 0]
  Constant5 : Constant  Value=[0 0 0]
  Constant6 : Constant  Commented=on  Value=[1 1]
  Mux : Mux  Inputs=6
  Selector : Selector  InputPortWidth=7  IndexOptions=Index vector (dialog)  Indices=[1 3]  OutputSizes=1
  uvec to Rvec : Subsystem
  road : Outport
  wires:
  Constant1/1 -> Bus Creator/1  "uvec"
  Constant2/1 -> Bus Creator/2  "gz"
  RdBus/1 -> Bus Selector/1
  Constant3/1 -> Mux/1
  Bus Selector/1 -> Mux/2  "<gz>"
  Mux/1 -> road/1
  Constant4/1 -> Mux/4
  Constant5/1 -> Mux/5
  Constant6/1 -> Bus Creator/3  "TyreScaling"
  Bus Selector/3 -> Selector/1  "<TyreScaling>"
  Bus Selector/2 -> uvec to Rvec/1(<uvec>)  "<uvec>"
  uvec to Rvec/1(Rvec) -> Mux/3
  Selector/1 -> Mux/6  "mu"

== system Tire_MFSwift/MFSwift/Road Inputs/Test Rig Post ==
  Moving Road : mfswift_simscape_library/Moving Road  response_time=0.05  tyre_id=100000
  Step road input 2 : Step  Time=4  After=0.05  SampleTime=0
  road : Outport
  wires:
  Moving Road/1 -> road/1
  Step road input 2/1 -> Moving Road/1

== system Tire_MFSwift/CPI Tire/Transform to Spin Frame CPI/Angle Fixed to Spinning/Get uvec Yaw axis ==
  note: Obtain unit vector along vertical axis within tire plane (wheel yaw axis)
      | (World Z vector [0 0 1])  -  (z-component of unit vector along wheel spin axis)
      | normalize ([0 0 1] - ([0 0 1].*uvec spin axis)*uvec spin axis)
  note: Make Unit Vector
  zf : Inport
  Add : Sum
  Constant : Constant
  Demux : Demux  Outputs=3
  Divide : Product  Inputs=*/
  Gain2 : Gain  Gain=-1
  Mult : Product  Inputs=**
  Mult1 : Product  Inputs=**
  Mult2 : Product  Inputs=**
  Mux1 : Mux  Inputs=3
  magnitude : Fcn  Expr=sqrt(u(1)*u(1)+u(2)*u(2)+u(3)*u(3))
  u : Outport
  wires:
  magnitude/1 -> Divide/2
  Divide/1 -> u/1
  Constant/1 -> Add/2
  Mult/1 -> Mux1/1
  Mult1/1 -> Mux1/2
  Gain2/1 -> Mult/2, Mult1/2, Mult2/2
  Demux/3 -> Mult2/1, Gain2/1
  zf/1 -> Demux/1
  Demux/1 -> Mult/1
  Mult2/1 -> Add/1
  Mux1/1 -> Divide/1, magnitude/1  "u0"
  Demux/2 -> Mult1/1
  Add/1 -> Mux1/3

== system Tire_MFSwift/MFSwift/Road Inputs/External Road/uvec to Rvec ==
  <uvec> : Inport
  Constant : Constant  Value=0
  Demux : Demux  Outputs=3
  Gain : Gain  Gain=-1
  Trigonometric Function1 : Trigonometry  Operator=atan2
  Trigonometric Function2 : Trigonometry  Operator=atan2
  YPR to Rvec : Subsystem
  Rvec : Outport
  wires:
  Trigonometric Function2/1 -> YPR to Rvec/2(pitch)  "Pitch"
  Gain/1 -> Trigonometric Function1/1
  Constant/1 -> YPR to Rvec/1(yaw)
  <uvec>/1 -> Demux/1
  YPR to Rvec/1(Rvec) -> Rvec/1
  Demux/3 -> Trigonometric Function2/2, Trigonometric Function1/2
  Demux/1 -> Trigonometric Function2/1
  Demux/2 -> Gain/1
  Trigonometric Function1/1 -> YPR to Rvec/3(roll)  "Roll"

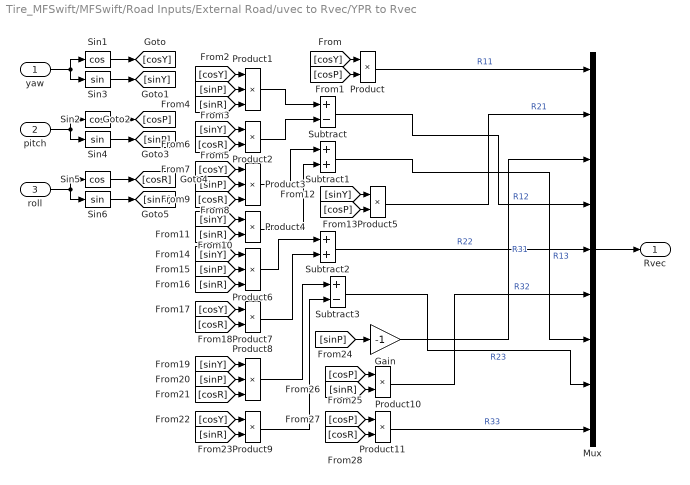
== system Tire_MFSwift/MFSwift/Road Inputs/External Road/uvec to Rvec/YPR to Rvec ==
  yaw : Inport
  pitch : Inport  Port=2
  roll : Inport  Port=3
  Gain : Gain  Gain=-1
  Mux : Mux  Inputs=9
  Product{,2,4..5,7,9..11} (8 alike) : Product
  Product{1,3,6,8} (4 alike) : Product  Inputs=3
  Sin1 : Trigonometry  Operator=cos
  Sin2 : Trigonometry  Operator=cos
  Sin3 : Trigonometry
  Sin4 : Trigonometry
  Sin5 : Trigonometry  Operator=cos
  Sin6 : Trigonometry
  Subtract : Sum  Inputs=+-
  Subtract1 : Sum
  Subtract2 : Sum
  Subtract3 : Sum  Inputs=+-
  Rvec : Outport  VectorParamsAs1DForOutWhenUnconnected=on
  wires:
  Sin4/1 -> [sinP]
  [sinP] -> Product6/2
  Product4/1 -> Subtract1/2
  [cosY] -> Product3/1
  Subtract3/1 -> Mux/8  "R23"
  [sinY] -> Product8/1
  Subtract2/1 -> Mux/5  "R22"
  [cosP] -> Product10/1
  [cosY] -> Product/1
  [sinP] -> Product3/2
  [sinY] -> Product2/1
  yaw/1 -> Sin1/1, Sin3/1
  Subtract/1 -> Mux/4  "R12"
  Sin2/1 -> [cosP]
  Sin5/1 -> [cosR]
  [cosR] -> Product11/2
  [sinP] -> Gain/1
  [sinR] -> Product10/2
  [sinR] -> Product1/3
  [cosR] -> Product8/3
  roll/1 -> Sin5/1, Sin6/1
  Product5/1 -> Mux/2  "R21"
  Product8/1 -> Subtract3/1
  Sin1/1 -> [cosY]
  [cosR] -> Product7/2
  Product11/1 -> Mux/9  "R33"
  Product1/1 -> Subtract/1
  [sinY] -> Product4/1
  [sinP] -> Product8/2
  [cosY] -> Product1/1
  [cosY] -> Product7/1
  Sin6/1 -> [sinR]
  Product2/1 -> Subtract/2
  [cosY] -> Product9/1
  [cosP] -> Product11/1
  [cosP] -> Product/2
  Product9/1 -> Subtract3/2
  [cosR] -> Product2/2
  [sinR] -> Product4/2
  Product/1 -> Mux/1  "R11"
  [sinY] -> Product5/1
  Product7/1 -> Subtract2/2
  [cosP] -> Product5/2
  Sin3/1 -> [sinY]
  Product10/1 -> Mux/6  "R32"
  [sinP] -> Product1/2
  [cosR] -> Product3/3
  Gain/1 -> Mux/3  "R31"
  Mux/1 -> Rvec/1
  pitch/1 -> Sin4/1, Sin2/1
  [sinY] -> Product6/1
  Subtract1/1 -> Mux/7  "R13"
  Product6/1 -> Subtract2/1
  [sinR] -> Product6/3
  [sinR] -> Product9/2
  Product3/1 -> Subtract1/1
